simulink model "Simulink_Regu"  (R2020b)
settings: Solver=VariableStepAuto  StartTime=0.0  StopTime=10.0  RelTol=1e-3
values from neighbouring files (symbols this model uses):
  A = pi    (= 3.14159265359)    [ControlNivel.m]
  h0 = 1.5    [ControlNivel.m]
  Ke = 0.25/10    (= 0.025)    [ControlNivel.m]
  Ks = 0.3543/(10*sqrt(3))    [ControlNivel.m]
  u20 = 5.0    (= 5)    [ControlNivel.m]
settings Model: Creator=serbogr1  LastModifiedBy=bou

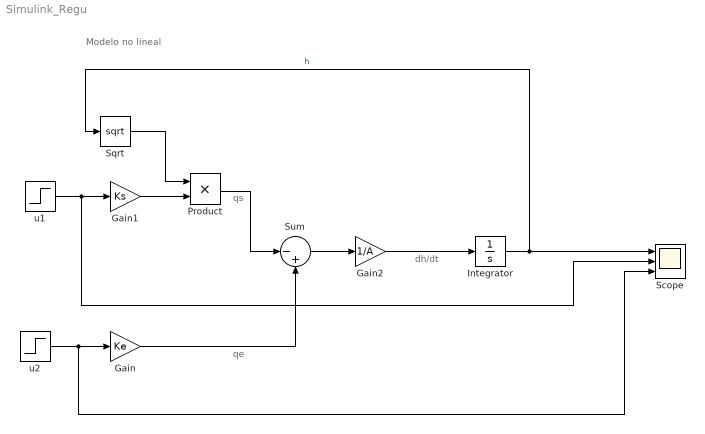
== system Simulink_Regu ==
  note: Modelo no lineal
  note: qe
  note: qs
  note: dh/dt
  Gain : Gain  Gain=Ke
  Gain1 : Gain  Gain=Ks
  Gain2 : Gain  Gain=1/A
  Integrator : Integrator
  Product : Product
  Scope : Scope  NumInputPorts=3
  Sqrt : Sqrt  SaturateOnIntegerOverflow=on
  Sum : Sum  Inputs=|-+
  "u1 " : Step  Before=Ke*u20/(Ks*sqrt(h0))  After=Ke*u20/(Ks*sqrt(h0))  SampleTime=0
  "u2 " : Step  Before=5.0  After=5.0  SampleTime=0
  wires:
  Gain/1 -> Sum/2
  "u2 "/1 -> Scope/3, Gain/1
  "u1 "/1 -> Scope/2, Gain1/1
  Gain1/1 -> Product/2
  Sqrt/1 -> Product/1
  Integrator/1 -> Sqrt/1, Scope/1  "h"
  Sum/1 -> Gain2/1
  Gain2/1 -> Integrator/1
  Product/1 -> Sum/1
